simulink model "opSpacePDControl"  (R2021b)
settings: Solver=VariableStepAuto  StartTime=0.0  StopTime=3  RelTol=1e-3
undefined symbols (not defined in the file): Kd, Kp, xd
settings Model: Creator=fabio  LastModifiedBy=buse

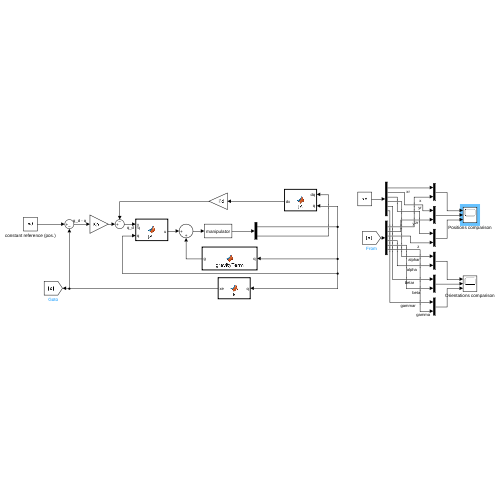
[thumbnail: Simulink's stored preview of the top-level diagram]
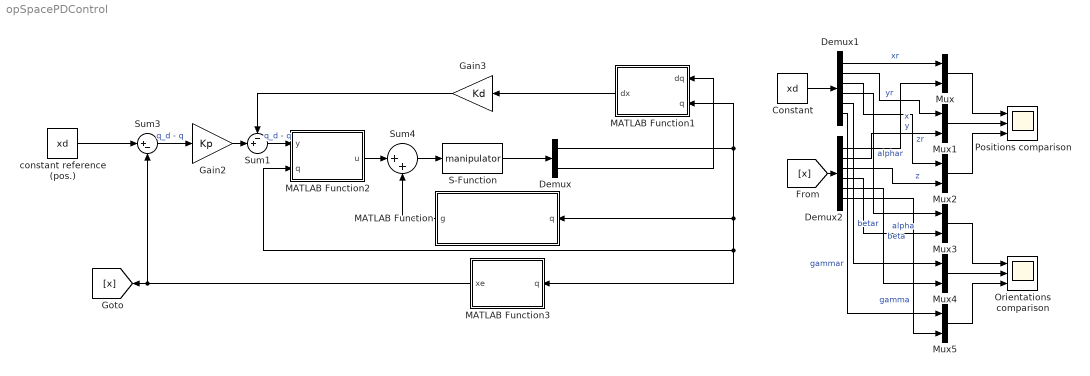
== system opSpacePDControl ==
  Constant : Constant  Value=xd
  Demux : Demux  Outputs=2
  Demux1 : Demux  Outputs=6
  Demux2 : Demux  Outputs=6
  Gain2 : Gain  Gain=Kp
  Gain3 : Gain  Gain=Kd
  MATLAB Function : MATLAB Function  TreatAsAtomicUnit=on
  MATLAB Function1 : MATLAB Function  TreatAsAtomicUnit=on
  MATLAB Function2 : MATLAB Function  TreatAsAtomicUnit=on
  MATLAB Function3 : MATLAB Function  TreatAsAtomicUnit=on
  Mux{,1..5} (6 alike) : Mux  Inputs=2
  Orientations comparison : Scope  NumInputPorts=3
  Positions comparison : Scope  NumInputPorts=3
  S-Function : S-Function  FunctionName=manipulator  Parameters=robot  SFunctionDeploymentMode=off  EnableBusSupport=off
  Sum1 : Sum  Inputs=-+|
  Sum3 : Sum  Inputs=|+-
  Sum4 : Sum  Inputs=|++
  constant reference (pos.) : Constant  Value=xd
  wires:
  Sum3/1 -> Gain2/1  "q_d - q"
  S-Function/1 -> Demux/1
  Demux/2 -> MATLAB Function1/1(dq)
  constant reference (pos.)/1 -> Sum3/1
  Demux/1 -> MATLAB Function2/2(q), MATLAB Function3/1(q), MATLAB Function/1(q), MATLAB Function1/2(q)
  MATLAB Function1/1(dx) -> Gain3/1
  Sum4/1 -> S-Function/1
  MATLAB Function3/1(xe) -> [x], Sum3/2
  MATLAB Function2/1(u) -> Sum4/1
  MATLAB Function/1(g) -> Sum4/2
  Gain2/1 -> Sum1/2
  Sum1/1 -> MATLAB Function2/1(y)  "q_d - q"
  Gain3/1 -> Sum1/1
  Demux2/5 -> Mux4/2  "beta"
  Demux2/4 -> Mux3/2  "alpha"
  Mux/1 -> Positions comparison/1
  Demux2/1 -> Mux/2  "x"
  Demux1/2 -> Mux1/1  "yr"
  Mux5/1 -> Orientations comparison/3
  Mux3/1 -> Orientations comparison/1
  Demux1/6 -> Mux5/1  "gammar"
  Demux1/4 -> Mux3/1  "alphar"
  Mux2/1 -> Positions comparison/3
  Demux2/3 -> Mux2/2  "z"
  Mux4/1 -> Orientations comparison/2
  Demux1/1 -> Mux/1  "xr"
  Demux1/5 -> Mux4/1  "betar"
  Demux1/3 -> Mux2/1  "zr"
  Demux2/2 -> Mux1/2  "y"
  Mux1/1 -> Positions comparison/2
  Demux2/6 -> Mux5/2  "gamma"
  Constant/1 -> Demux1/1
  [x] -> Demux2/1

== matlab function opSpacePDControl/MATLAB Function1 ==
  data: dq input; dx output; q input
function dx = JA(dq, q)
    q1 = q(1); q2 = q(2); q3 = q(3);
    JA =[(3*cos(q1))/10 - (2*sin(q1))/5 + (6*cos(q1)*cos(q3))/25 + q2*cos(q1),  sin(q1), -(6*sin(q1)*sin(q3))/25;
        (2*cos(q1))/5 + (3*sin(q1))/10 + (6*cos(q3)*sin(q1))/25 + q2*sin(q1), -cos(q1),  (6*cos(q1)*sin(q3))/25;
        0,        0,          (6*cos(q3))/25;
        1,        0,                       0;
        0,        0,                      -1;
        0,        0,                       0]; 
    dx = JA*dq;

== matlab function opSpacePDControl/MATLAB Function ==
  data: q input; g output
function g = gravityTerm(q)  
       g = [      0;
             0;
0.9621*cos(q(3))];
end

== matlab function opSpacePDControl/MATLAB Function2 ==
  data: y input; u output; q input
function u = JAT(y, q)
    q1 = q(1); q2 = q(2); q3 = q(3);
    JA =[(3*cos(q1))/10 - (2*sin(q1))/5 + (6*cos(q1)*cos(q3))/25 + q2*cos(q1),  sin(q1), -(6*sin(q1)*sin(q3))/25;
        (2*cos(q1))/5 + (3*sin(q1))/10 + (6*cos(q3)*sin(q1))/25 + q2*sin(q1), -cos(q1),  (6*cos(q1)*sin(q3))/25;
        0,        0,          (6*cos(q3))/25;
        1,        0,                       0;
        0,        0,                      -1;
        0,        0,                       0]; 
    u = JA'*y;

== matlab function opSpacePDControl/MATLAB Function3 ==
  data: q input size=3; xe output size=6
function xe = k(q)
    q1 = q(1); q2 = q(2); q3 = q(3);
    % Direct kinematics
    xe = [(2*cos(q1))/5 + (3*sin(q1))/10 + (6*cos(q3)*sin(q1))/25 + q2*sin(q1);
         (2*sin(q1))/5 - (3*cos(q1))/10 - (6*cos(q1)*cos(q3))/25 - q2*cos(q1);
         (6*sin(q3))/25 + 3/20;
         q1;
         pi/2 - q3;
         pi/2];
